simulink model "Facilitation"  (Simulink 6.3)
settings: Solver=ode23s  StartTime=0  StopTime=300  MaxStep=0.01  RelTol=1e-3
undefined symbols (not defined in the file or in its folder): sigbuilder_block
Description:
  | This is a model of depression in synapses
settings Model: Creator=chchlee  LastModifiedBy=Owner  ExtModeAutoUpdateStatusClock=off
settings DataIOCC: SignalLoggingName=sigsOut
settings OptimizationCC: InlineInvariantSignals=on
settings DebuggingCC: SolverPrmCheckMsg=none
settings HardwareCC: TargetUnknown=on
settings GRTTargetCC: ModelReferenceCompliant=off  MatFileLogging=off

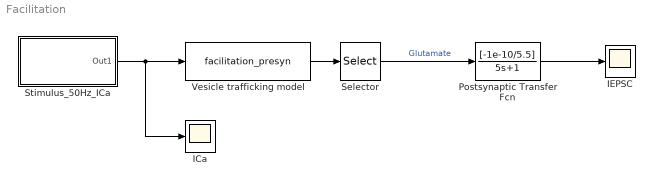
== system Facilitation ==
  ICa : Scope
      settings: YMin=-67.5  YMax=-63  SaveName=ScopeData3
  IEPSC : Scope
      settings: YMin=-8e-007  YMax=0  SaveName=sim_facilitation  DataFormat=Array
  Postsynaptic Transfer Fcn : TransferFcn  Numerator=[-1e-10/5.5]  Denominator=[5 1]
  Selector : Selector  Elements=[4]  InputPortWidth=4
  Stimulus_50Hz_ICa : Subsystem
  Vesicle trafficking model : S-Function  FunctionName=facilitation_presyn
  wires:
  Selector/1 -> Postsynaptic Transfer Fcn/1  "Glutamate"
  Vesicle trafficking model/1 -> Selector/1
  Stimulus_50Hz_ICa/1(Out1) -> ICa/1, Vesicle trafficking model/1
  Postsynaptic Transfer Fcn/1 -> IEPSC/1

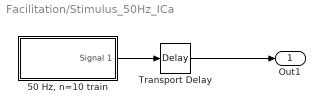
== system Facilitation/Stimulus_50Hz_ICa ==
  "50 Hz, n=10 train" : Subsystem  Tag=STV Subsys  LoadFcn=sigbuilder_block('load');  StartFcn=sigbuilder_block('start');  StopFcn=sigbuilder_block('stop');  ClipboardFcn=sigbuilder_block('clipboard');  mask(Sigbuilder block){}
      mask help: Sigbuilder GUI
      mask init:
      | if ~strcmp(get_param(bdroot(gcbh),'SimulationStatus'),'stopped') tuvar = sigbuilder_block('maskInit'); end
      settings: CopyFcn=sigbuilder_block('copy');  DeleteFcn=sigbuilder_block('delete');  ModelCloseFcn=sigbuilder_block('modelClose');  PreSaveFcn=sigbuilder_block('preSave');  NameChangeFcn=sigbuilder_block('namechange');  OpenFcn=sigbuilder_block('open',[-1.5 5.25 768 498 ]);  CloseFcn=sigbuilder_block('close');
      mask Display: plot(0,0,100,100,[10,10,40,40,10],[80,20,20,80,80],[40,10],[50,50], [40,27,10],[65,72,56],[40,25,25,10],[28,28,43,43]);
  Transport Delay : TransportDelay  DelayTime=11.5  BufferSize=2000
  Out1 : Outport
  wires:
  Transport Delay/1 -> Out1/1
  "50 Hz, n=10 train"/1(Signal 1) -> Transport Delay/1

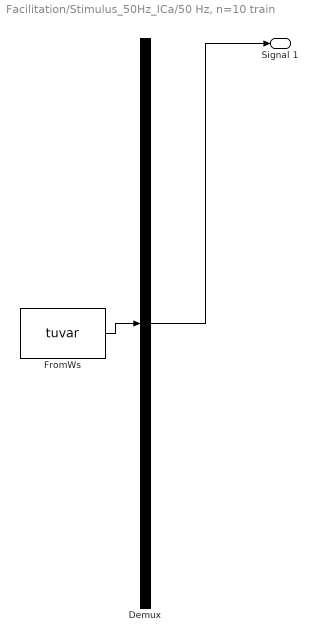
== system Facilitation/Stimulus_50Hz_ICa/50 Hz, n=10 train ==
  Demux : Demux  Tag=STV Demux  Outputs=1
  FromWs : FromWorkspace  Tag=STV FromWs  VariableName=tuvar  SampleTime=0  SigBuilderData=DataTag0  VnvData=DataTag1
      SigBuilderData=|
      | channels.label = 'Signal 1'
      | channels.allXData = {[0 1 1 20 20 21 21 40 40 41 41 60 60 61 61 80 80 81 81 100 100 101 101 120 120 121 121 140 140 141 141 160 160 161 161 180 180 181 181 200 250]}
      | channels.allYData = {[1 1 0 0 1 1 0 0 1 1 0 0 1 1 0 0 1 1 0 0 1 1 0 0 1 1 0 0 1 1 0 0 1 1 0 0 1 1 0 0 0]}
      | dataSet.timeRange = [0 250]
      | dataSet.name = 'Group 1'
  Signal 1 : Outport  Tag=STV Outport
  wires:
  Demux/1 -> Signal 1/1
  FromWs/1 -> Demux/1
